simulink subsystem "InverterLogic"  (R2024b)
settings: Solver=VariableStepAuto  StartTime=0.0  StopTime=10.0  RelTol=1e-3
settings Model: Creator=luigi  LastModifiedBy=luigi

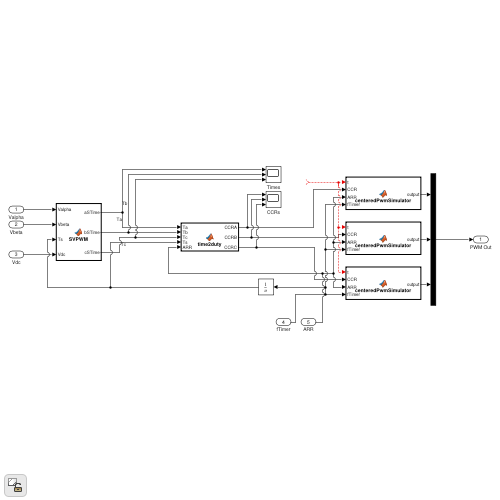
[thumbnail: Simulink's stored preview of the top-level diagram]
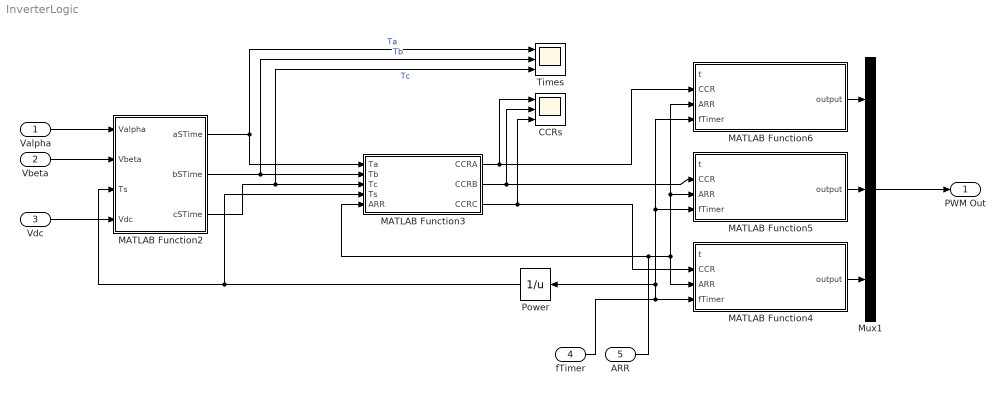
== system InverterLogic ==
  Valpha : Inport
  Vbeta : Inport  Port=2
  Vdc : Inport  Port=3
  fTimer : Inport  Port=4
  ARR : Inport  Port=5
  CCRs : Scope  NumInputPorts=3
  MATLAB Function2 : MATLAB Function  TreatAsAtomicUnit=on
  MATLAB Function3 : MATLAB Function  TreatAsAtomicUnit=on
  MATLAB Function4 : MATLAB Function  TreatAsAtomicUnit=on
  MATLAB Function5 : MATLAB Function  TreatAsAtomicUnit=on
  MATLAB Function6 : MATLAB Function  TreatAsAtomicUnit=on
  Mux1 : Mux  Inputs=3
  Power : Math  Operator=reciprocal
  Times : Scope  NumInputPorts=3
  PWM Out : Outport
  wires:
  MATLAB Function3/3(CCRC) -> CCRs/3, MATLAB Function4/2(CCR)
  MATLAB Function2/3(cSTime) -> MATLAB Function3/3(Tc), Times/3  "Tc"
  Valpha/1 -> MATLAB Function2/1(Valpha)
  Vbeta/1 -> MATLAB Function2/2(Vbeta)
  MATLAB Function6/1(output) -> Mux1/1
  MATLAB Function2/2(bSTime) -> MATLAB Function3/2(Tb), Times/2  "Tb"
  fTimer/1 -> MATLAB Function4/4(fTimer), Power/1, MATLAB Function6/4(fTimer), MATLAB Function5/4(fTimer)
  MATLAB Function5/1(output) -> Mux1/2
  MATLAB Function2/1(aSTime) -> Times/1, MATLAB Function3/1(Ta)  "Ta"
  MATLAB Function3/2(CCRB) -> CCRs/2, MATLAB Function5/2(CCR)
  Power/1 -> MATLAB Function3/4(Ts), MATLAB Function2/3(Ts)
  ARR/1 -> MATLAB Function3/5(ARR), MATLAB Function6/3(ARR), MATLAB Function5/3(ARR), MATLAB Function4/3(ARR)
  Mux1/1 -> PWM Out/1
  MATLAB Function4/1(output) -> Mux1/3
  ? -> MATLAB Function6/1(t), MATLAB Function4/1(t), MATLAB Function5/1(t)
  Vdc/1 -> MATLAB Function2/4(Vdc)
  MATLAB Function3/1(CCRA) -> MATLAB Function6/2(CCR), CCRs/1

== matlab function InverterLogic/MATLAB Function2 ==
  data: Valpha input; aSTime output; Vbeta input; Ts input; Vdc input; bSTime output; cSTime output
function [aSTime, bSTime, cSTime] = SVPWM(Valpha, Vbeta, Ts, Vdc)
Ts = Ts./2;

piThird = pi/3;
scaling = 2/sqrt(3);


% First step: determine the angle of the reference
if(Valpha == 0)
    theta = 0;
else
    theta = atan(Vbeta/Valpha);
end

if(theta < 0)
    theta = theta + pi;
end

if(Vbeta < 0)
    theta = theta + pi;
end

Vref = sqrt(Valpha*Valpha+Vbeta*Vbeta);

quad = floor(theta/piThird) + 1;

modulation = (3/2) * (Vref/Vdc);

ThB = (quad-1) * piThird; %Angle of first possible vector
ThA = quad * piThird; %Angle of the second vector

Ta = scaling * modulation * Ts * sin(ThA - theta);
Tb = scaling * modulation * Ts * sin(theta - ThB);
Tz = Ts - Ta - Tb;

aSTime = 0;
bSTime = 0;
cSTime = 0;

switch quad
    case 1
        aSTime = Ta + Tb + Tz/2;
        bSTime = Tb + Tz/2;
        cSTime = Tz/2;
    case 2
        aSTime = Ta + Tz/2;
        bSTime  = Ta + Tb + Tz/2;
        cSTime  = Tz/2;
    case 3
        aSTime = Tz/2;
        bSTime = Ta + Tb + Tz/2;
        cSTime  = Tb + Tz/2;
    case 4
        aSTime = Tz/2;
        bSTime = Ta + Tz/2;
        cSTime  = Ta + Tb + Tz/2;
    case 5
        aSTime = Tb + Tz/2;
        bSTime = Tz/2;
        cSTime = Ta + Tb + Tz/2;
    case 6
        aSTime  = Ta + Tb + Tz/2;
        bSTime = Tz/2;
        cSTime = Ta + Tz/2;
    otherwise
        error("Invalid quadrant in SVPWM");
end

== matlab function InverterLogic/MATLAB Function3 ==
  data: Ta input; Tb input; Tc input; CCRA output; Ts input; CCRB output; CCRC output; ARR input
function [CCRA, CCRB, CCRC] = time2duty(Ta, Tb, Tc, Ts, ARR)
% This function converts switching times to CCR values for timers
% set in PWM Mode 3 - Center Aligned

dcA = Ta / Ts;
dcB = Tb / Ts;
dcC = Tc / Ts;

% CCRA / ARR = dcA;
CCRA = ARR * (1-dcA);
CCRB = ARR * (1-dcB);
CCRC = ARR * (1-dcC);
end

== matlab function InverterLogic/MATLAB Function4 ==
  settings: updateMethod=DISCRETE
  data: t input; output output; CCR input; ARR input; fTimer input
function output  = centeredPwmSimulator(t, CCR, ARR, fTimer)
% This function aims to emulate the behaviour of a single channel
% of the STM32 PWM hardware 

Ts = 1/fTimer;

persistent counter
persistent timeCounter
persistent direction
persistent outState
if isempty(outState)
    outState = 0;
end
if isempty(timeCounter)
    timeCounter = 0;
end
if isempty(counter)
    counter = 0;
end
if isempty(direction)
    direction = 1;
end

if (t - timeCounter * Ts) > 0
    delta = 1;
    timeCounter = timeCounter + 1;
else 
    delta = 0;
end

if counter >= ARR
    direction = -1;
end
if counter <= 0
    direction = 1;
end

counter = counter + delta .* direction;

if(counter == round(CCR) && delta ~= 0)
    if(outState == 0)
        outState = 1;
    else
        outState = 0;
    end
end

output = outState;

end

== matlab function InverterLogic/MATLAB Function5 ==
  settings: updateMethod=DISCRETE
  data: t input; output output; CCR input; ARR input; fTimer input
function output  = centeredPwmSimulator(t, CCR, ARR, fTimer)
% This function aims to emulate the behaviour of a single channel
% of the STM32 PWM hardware 

Ts = 1/fTimer;

persistent counter
persistent timeCounter
persistent direction
persistent outState
if isempty(outState)
    outState = 0;
end
if isempty(timeCounter)
    timeCounter = 0;
end
if isempty(counter)
    counter = 0;
end
if isempty(direction)
    direction = 1;
end

if (t - timeCounter * Ts) > 0
    delta = 1;
    timeCounter = timeCounter + 1;
else 
    delta = 0;
end

if counter >= ARR
    direction = -1;
end
if counter <= 0
    direction = 1;
end

counter = counter + delta .* direction;

if(counter == round(CCR) && delta ~= 0)
    if(outState == 0)
        outState = 1;
    else
        outState = 0;
    end
end

output = outState;

end

== matlab function InverterLogic/MATLAB Function6 ==
  settings: updateMethod=DISCRETE
  data: t input; output output; CCR input; ARR input; fTimer input
function output  = centeredPwmSimulator(t, CCR, ARR, fTimer)
% This function aims to emulate the behaviour of a single channel
% of the STM32 PWM hardware 

Ts = 1/fTimer;

persistent counter
persistent timeCounter
persistent direction
persistent outState
if isempty(outState)
    outState = 0;
end
if isempty(timeCounter)
    timeCounter = 0;
end
if isempty(counter)
    counter = 0;
end
if isempty(direction)
    direction = 1;
end

if (t - timeCounter * Ts) > 0
    delta = 1;
    timeCounter = timeCounter + 1;
else 
    delta = 0;
end

if counter >= ARR
    direction = -1;
end
if counter <= 0
    direction = 1;
end

counter = counter + delta .* direction;

if(counter == round(CCR) && delta ~= 0)
    if(outState == 0)
        outState = 1;
    else
        outState = 0;
    end
end

output = outState;

end
